simulink model "threeLinks_opt_joint_limit"  (R2016b)
settings: Solver=FixedStepDiscrete  StartTime=0.0  StopTime=inf  FixedStep=Ts  RelTol=1e-3  EnableMultiTasking=on
StartFcn:
  | foundFig=findobj('Tag','trajScope');
  | if ~isempty(foundFig)
  |    close(foundFig);
  | end
undefined symbols (not defined in the file): DiscIntNeverNeededParam, Ts
libraries: simulink x3
settings Model: Creator=pattacini  LastModifiedBy=ben
settings DataIOCC: SaveFormat=Array  SignalLoggingSaveFormat=ModelDataLogs  SaveOutput=off  SignalLogging=off  SaveTime=off
settings OptimizationCC: ExpressionDepthLimit=2147483647  LifeSpan=inf
settings DebuggingCC: UnderspecifiedInitializationDetection=Classic  MergeDetectMultiDrivingBlocksExec=none  SolverPrmCheckMsg=warning  FcnCallInpInsideContextMsg=warning  StateNameClashWarn=warning  SFUnexpectedBacktrackingDiag=warning  SFNoUnconditionalDefaultTransitionDiag=warning  SFExecutionAtInitializationDiag=none
settings HardwareCC: ProdBitPerPointer=32  ProdBitPerSizeT=32  ProdBitPerPtrDiffT=32  ProdLargestAtomicFloat=None  ProdIntDivRoundTo=Undefined  ProdEndianess=Unspecified  ProdWordSize=32  ProdHWDeviceType=32-bit Generic
settings ModelReferenceCC: PropagateSignalLabelsOutOfModel=off
settings SFSimCC: SimParseCustomCode=off
settings GRTTargetCC: TargetLangStandard=C89/C90 (ANSI)  CombineOutputUpdateFcns=off  GRTInterface=on
settings ConfigComp: CovMetricSettings=dw  CovHtmlReporting=on  CovSaveCumulativeToWorkspaceVar=on  CovSaveSingleToWorkspaceVar=on  CovExternalEMLEnable=off

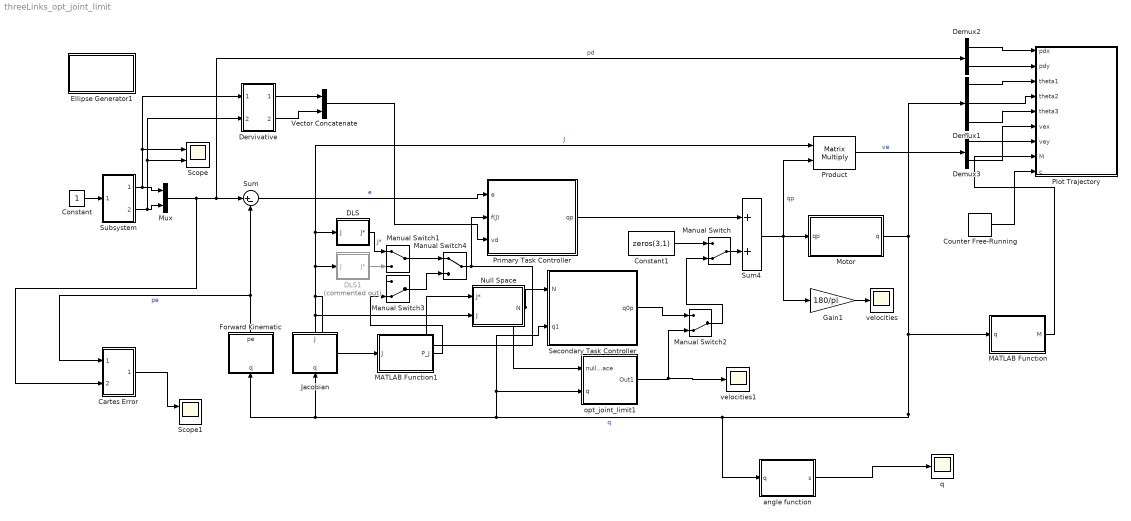
== system threeLinks_opt_joint_limit ==
  Cartes Error : Subsystem
  Constant : Constant
  Constant1 : Constant  Value=zeros(3,1)
  Counter Free-Running : simulink/Sources/Counter Free-Running  NumBits=16  tsamp=-1
  DLS : Subsystem  mask(Motor settings){k=0.01}
      mask Display: port_label('input',1,'DLS');
  DLS1 : Subsystem  Commented=on  mask(Motor settings){W=[4 0 0; 0 1 0; 0 0 1]}
      mask prompts: W "W matrix(3*3)"
      mask Display: port_label('input',1,'W J*');
  Demux1 : Demux  Outputs=3
  Demux2 : Demux  Outputs=2
  Demux3 : Demux  Outputs=2
  Dervivative : Subsystem
  Ellipse Generator1 : Subsystem  mask(Edit sample time){Ts=0.01}
      mask prompts: Ts "Ts [s]:"
      mask init:
      | assignin('base','Ts',Ts);
      mask Display: disp('Edit\nSample Time');
  Forward Kinematic : Subsystem
  Gain1 : Gain  Gain=180/pi
  Jacobian : Subsystem
  MATLAB Function : MATLAB Function  TreatAsAtomicUnit=on
  MATLAB Function1 : MATLAB Function  TreatAsAtomicUnit=on
  Manual Switch : ManualSwitch  CurrentSetting=0
  Manual Switch1 : ManualSwitch
  Manual Switch2 : ManualSwitch  CurrentSetting=0
  Manual Switch3 : ManualSwitch  CurrentSetting=0
  Manual Switch4 : ManualSwitch
  Motor : Subsystem  mask(Motor settings){q0=[pi/4;  pi/4 ;  -pi/4]}
      mask prompts: q0 "Initial position [2x1]:"
      mask Display:
      | disp('Motor');
      | port_label('input',1,'qp');
      | port_label('output',1,'q');
  Mux : Mux  Inputs=2
      settings: DisplayOption=signals
  Null Space : Subsystem
  Plot Trajectory : MATLAB Function  TreatAsAtomicUnit=on
  Primary Task Controller : Subsystem  mask(Controller settings){K=[50 0; 0 50]}
      mask prompts: K "Gain matrix [2x2]:"
      mask Display: disp('qp=J**K*e');
  Product : Product  Multiplication=Matrix(*)  RndMeth=Zero
  Scope : Scope  NumInputPorts=2
  Scope1 : Scope  NumInputPorts=2
  Secondary Task Controller : Subsystem  mask(Controller settings){k=[0 0 1]', q0=[0 0 0]'}
  Subsystem : Subsystem
      mask Display: disp('Input Signal')
  Sum : Sum  Inputs=|+-
  Sum4 : Sum  Inputs=2
  Vector Concatenate : Concatenate
  "angle function " : MATLAB Function  TreatAsAtomicUnit=on
  opt_joint_limit1 : Subsystem  mask{q_min=[-pi;-pi;-pi], q_max=[pi;pi;pi]}
      mask Display: disp('Secondary Task')
  "q " : Scope
  velocities : Scope
  velocities1 : Scope
  wires:
  Jacobian/1(J) -> MATLAB Function1/1(J), DLS1/1(J), Product/1, DLS/1(J), Null Space/2(J)  "J"
  Sum/1 -> Primary Task Controller/1(e)  "e"
  Forward Kinematic/1(pe) -> Cartes Error/1(In1), Sum/2  "pe"
  Mux/1 -> Cartes Error/2(In2), Sum/1, Demux2/1  "pd"
  Sum4/1 -> Product/2, Gain1/1, Motor/1(qp)  "qp"
  Motor/1(q) -> Demux1/1, "angle function "/1(q), opt_joint_limit1/2(q), Secondary Task Controller/2(q1), Forward Kinematic/1(q), Jacobian/1(q), MATLAB Function/1(q)  "q"
  Demux2/1 -> Plot Trajectory/1(pdx)
  Demux2/2 -> Plot Trajectory/2(pdy)
  Demux1/1 -> Plot Trajectory/3(theta1)
  Demux1/2 -> Plot Trajectory/4(theta2)
  Demux3/1 -> Plot Trajectory/6(vex)
  Demux3/2 -> Plot Trajectory/7(vey)
  Product/1 -> Demux3/1  "ve"
  Gain1/1 -> velocities/1
  Demux1/3 -> Plot Trajectory/5(theta3)
  Primary Task Controller/1(qp) -> Sum4/1
  Manual Switch/1 -> Sum4/2
  Constant1/1 -> Manual Switch/1
  Constant/1 -> Subsystem/1(In1)
  Subsystem/1(Out1) -> Dervivative/1(In1), Scope/1, Mux/1
  Subsystem/2(Out2) -> Dervivative/2(In2), Scope/2, Mux/2
  Dervivative/1(Out1) -> Vector Concatenate/1
  Dervivative/2(Out2) -> Vector Concatenate/2
  Vector Concatenate/1 -> Primary Task Controller/3(vd)
  DLS1/1(J*) -> Manual Switch1/2
  DLS/1(J*) -> Manual Switch1/1  "J*"
  Cartes Error/1(Out2) -> Scope1/1
  Null Space/1(N) -> opt_joint_limit1/1(nullspace), Secondary Task Controller/1(N)
  Secondary Task Controller/1(q0p) -> Manual Switch2/1
  Manual Switch2/1 -> Manual Switch/2
  MATLAB Function/1(M) -> Plot Trajectory/8(M)
  Counter Free-Running/1 -> Plot Trajectory/9(c)
  opt_joint_limit1/1(Out1) -> velocities1/1, Manual Switch2/2
  "angle function "/1(s) -> "q "/1
  MATLAB Function1/1(P_J) -> Manual Switch3/2
  Manual Switch3/1 -> Manual Switch4/2
  Manual Switch1/1 -> Manual Switch4/1
  Manual Switch4/1 -> Primary Task Controller/2(f(J)), Null Space/1(J*)

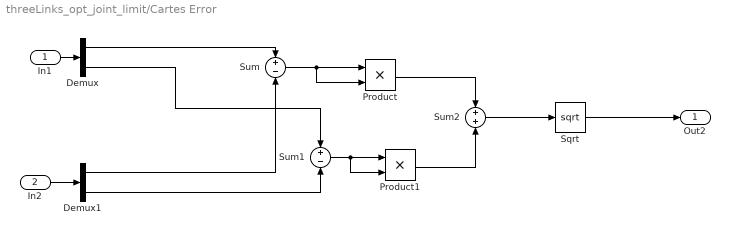
== system threeLinks_opt_joint_limit/Cartes Error ==
  In1 : Inport
  In2 : Inport  Port=2
  Demux : Demux  Outputs=2
  Demux1 : Demux  Outputs=2
  Product : Product
  Product1 : Product
  Sqrt : Sqrt  SaturateOnIntegerOverflow=on
  Sum : Sum  Inputs=+-
  Sum1 : Sum  Inputs=+-
  Sum2 : Sum
  Out2 : Outport
  wires:
  In1/1 -> Demux/1
  In2/1 -> Demux1/1
  Demux/1 -> Sum/1
  Demux1/1 -> Sum/2
  Demux/2 -> Sum1/1
  Demux1/2 -> Sum1/2
  Sum/1 -> Product/2, Product/1
  Sum1/1 -> Product1/2, Product1/1
  Product/1 -> Sum2/1
  Product1/1 -> Sum2/2
  Sum2/1 -> Sqrt/1
  Sqrt/1 -> Out2/1

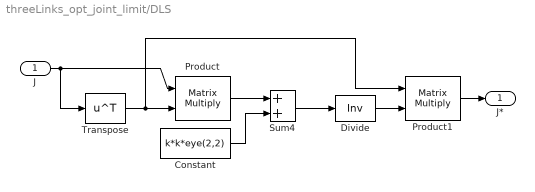
== system threeLinks_opt_joint_limit/DLS ==
  J : Inport
  Constant : Constant  Value=k*k*eye(2,2)
  Divide : Product  Inputs=/  Multiplication=Matrix(*)
  Product : Product  Multiplication=Matrix(*)  RndMeth=Zero
  Product1 : Product  Multiplication=Matrix(*)  RndMeth=Zero
  Sum4 : Sum
  Transpose : Math  Operator=transpose  SaturateOnIntegerOverflow=on
  J* : Outport
  wires:
  J/1 -> Transpose/1, Product/1
  Transpose/1 -> Product/2, Product1/1
  Product/1 -> Sum4/1
  Sum4/1 -> Divide/1
  Divide/1 -> Product1/2
  Product1/1 -> J*/1
  Constant/1 -> Sum4/2

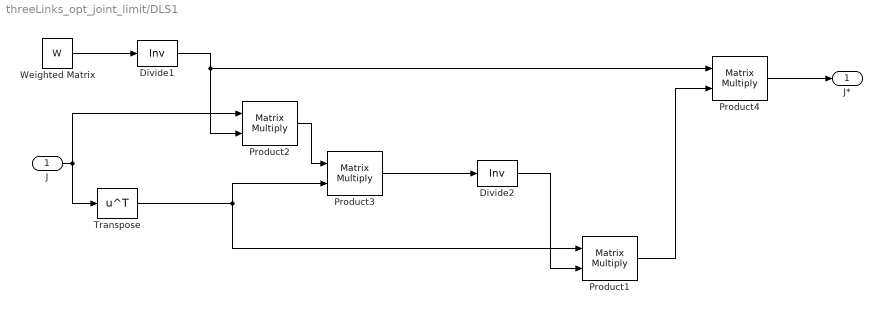
== system threeLinks_opt_joint_limit/DLS1 ==
  J : Inport
  Divide1 : Product  Inputs=/  Multiplication=Matrix(*)
  Divide2 : Product  Inputs=/  Multiplication=Matrix(*)
  Product{1..4} (4 alike) : Product  Multiplication=Matrix(*)  RndMeth=Zero
  Transpose : Math  Operator=transpose  SaturateOnIntegerOverflow=on
  Weighted Matrix : Constant  Value=W
  J* : Outport
  wires:
  J/1 -> Transpose/1, Product2/1
  Weighted Matrix/1 -> Divide1/1
  Divide1/1 -> Product2/2, Product4/1
  Transpose/1 -> Product1/1, Product3/2
  Product2/1 -> Product3/1
  Product3/1 -> Divide2/1
  Product4/1 -> J*/1
  Divide2/1 -> Product1/2
  Product1/1 -> Product4/2

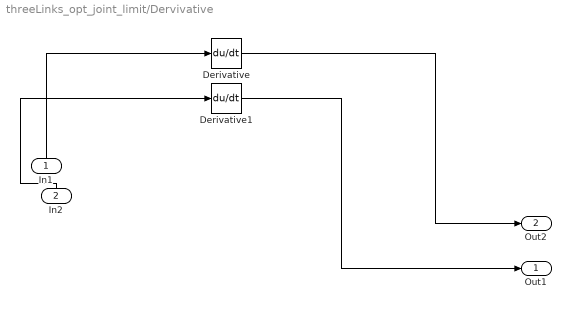
== system threeLinks_opt_joint_limit/Dervivative ==
  In1 : Inport
  In2 : Inport  Port=2
  Derivative : Derivative
  Derivative1 : Derivative
  Out1 : Outport
  Out2 : Outport  Port=2
  wires:
  Derivative/1 -> Out2/1
  In1/1 -> Derivative/1
  Derivative1/1 -> Out1/1
  In2/1 -> Derivative1/1

== system threeLinks_opt_joint_limit/Ellipse Generator1 ==

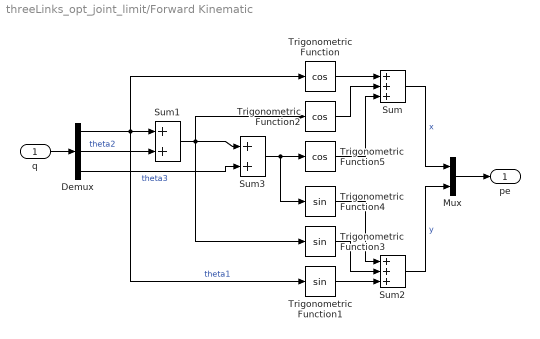
== system threeLinks_opt_joint_limit/Forward Kinematic ==
  q : Inport
  Demux : Demux  Outputs=3
  Mux : Mux  Inputs=2
  Sum : Sum  Inputs=3
  Sum1 : Sum
  Sum2 : Sum  Inputs=3
  Sum3 : Sum
  Trigonometric Function : Trigonometry  Operator=cos
  Trigonometric Function1 : Trigonometry
  Trigonometric Function2 : Trigonometry  Operator=cos
  Trigonometric Function3 : Trigonometry
  Trigonometric Function4 : Trigonometry
  Trigonometric Function5 : Trigonometry  Operator=cos
  pe : Outport
  wires:
  q/1 -> Demux/1
  Demux/1 -> Trigonometric Function1/1, Trigonometric Function/1, Sum1/1  "theta1"
  Mux/1 -> pe/1
  Sum1/1 -> Trigonometric Function2/1, Trigonometric Function3/1, Sum3/1
  Demux/2 -> Sum1/2  "theta2"
  Trigonometric Function1/1 -> Sum2/3
  Trigonometric Function3/1 -> Sum2/2
  Trigonometric Function/1 -> Sum/1
  Trigonometric Function2/1 -> Sum/2
  Demux/3 -> Sum3/2  "theta3"
  Sum3/1 -> Trigonometric Function5/1, Trigonometric Function4/1
  Trigonometric Function5/1 -> Sum/3
  Trigonometric Function4/1 -> Sum2/1
  Sum/1 -> Mux/1  "x"
  Sum2/1 -> Mux/2  "y"

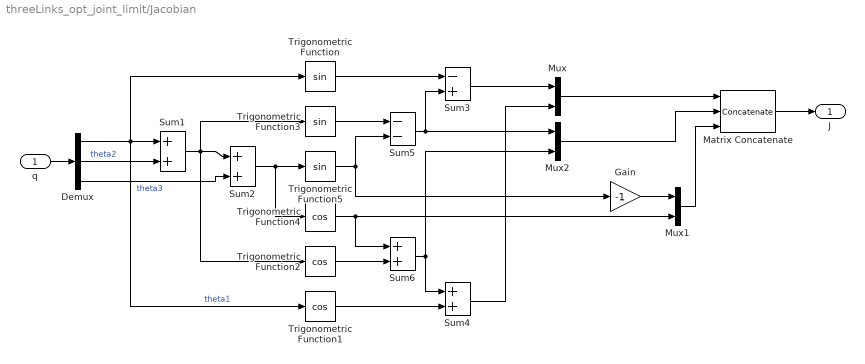
== system threeLinks_opt_joint_limit/Jacobian ==
  q : Inport
  Demux : Demux  Outputs=3
  Gain : Gain  Gain=-1
  Matrix Concatenate : Concatenate  NumInputs=3  Mode=Multidimensional array  ConcatenateDimension=2
  Mux : Mux  Inputs=2
  Mux1 : Mux  Inputs=2
  Mux2 : Mux  Inputs=2
  Sum1 : Sum
  Sum2 : Sum
  Sum3 : Sum  Inputs=-+
  Sum4 : Sum  Inputs=2
  Sum5 : Sum  Inputs=--
  Sum6 : Sum  Inputs=2
  Trigonometric Function : Trigonometry
  Trigonometric Function1 : Trigonometry  Operator=cos
  Trigonometric Function2 : Trigonometry  Operator=cos
  Trigonometric Function3 : Trigonometry
  Trigonometric Function4 : Trigonometry  Operator=cos
  Trigonometric Function5 : Trigonometry
  J : Outport
  wires:
  Demux/1 -> Trigonometric Function/1, Trigonometric Function1/1, Sum1/1  "theta1"
  q/1 -> Demux/1
  Matrix Concatenate/1 -> J/1
  Demux/2 -> Sum1/2  "theta2"
  Sum1/1 -> Trigonometric Function2/1, Trigonometric Function3/1, Sum2/1
  Gain/1 -> Mux1/1
  Demux/3 -> Sum2/2  "theta3"
  Sum2/1 -> Trigonometric Function5/1, Trigonometric Function4/1
  Sum3/1 -> Mux/1
  Sum4/1 -> Mux/2
  Trigonometric Function3/1 -> Sum5/1
  Trigonometric Function5/1 -> Gain/1, Sum5/2
  Sum5/1 -> Sum3/2, Mux2/1
  Trigonometric Function/1 -> Sum3/1
  Trigonometric Function2/1 -> Sum6/2
  Trigonometric Function4/1 -> Mux1/2, Sum6/1
  Trigonometric Function1/1 -> Sum4/2
  Sum6/1 -> Sum4/1, Mux2/2
  Mux/1 -> Matrix Concatenate/1
  Mux2/1 -> Matrix Concatenate/2
  Mux1/1 -> Matrix Concatenate/3

== system threeLinks_opt_joint_limit/Motor ==
  qp : Inport
  Discrete-Time Integrator : DiscreteIntegrator  IntegratorMethod=Integration: Trapezoidal  InitialCondition=q0  SampleTime=Ts  ICPrevOutput=DiscIntNeverNeededParam  ICPrevScaledInput=DiscIntNeverNeededParam
  Unit Delay : UnitDelay  InitialCondition=q0  SampleTime=-1
  q : Outport
  wires:
  qp/1 -> Discrete-Time Integrator/1
  Discrete-Time Integrator/1 -> Unit Delay/1
  Unit Delay/1 -> q/1

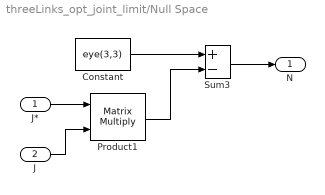
== system threeLinks_opt_joint_limit/Null Space ==
  J* : Inport
  J : Inport  Port=2
  Constant : Constant  Value=eye(3,3)
  Product1 : Product  Multiplication=Matrix(*)  RndMeth=Zero
  Sum3 : Sum  Inputs=+-
  N : Outport
  wires:
  J*/1 -> Product1/1
  J/1 -> Product1/2
  Constant/1 -> Sum3/1
  Product1/1 -> Sum3/2
  Sum3/1 -> N/1

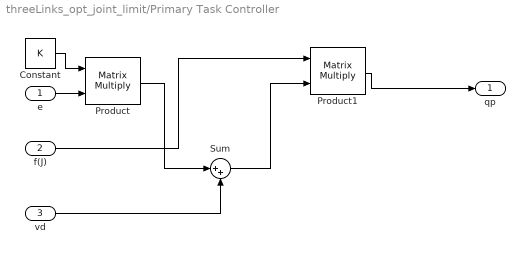
== system threeLinks_opt_joint_limit/Primary Task Controller ==
  e : Inport
  f(J) : Inport  Port=2
  vd : Inport  Port=3
  Constant : Constant  Value=K
  Product : Product  Multiplication=Matrix(*)  RndMeth=Zero
  Product1 : Product  Multiplication=Matrix(*)  RndMeth=Zero
  Sum : Sum  Inputs=|++
  qp : Outport
  wires:
  f(J)/1 -> Product1/1
  e/1 -> Product/2
  Constant/1 -> Product/1
  Product/1 -> Sum/1
  Product1/1 -> qp/1
  vd/1 -> Sum/2
  Sum/1 -> Product1/2

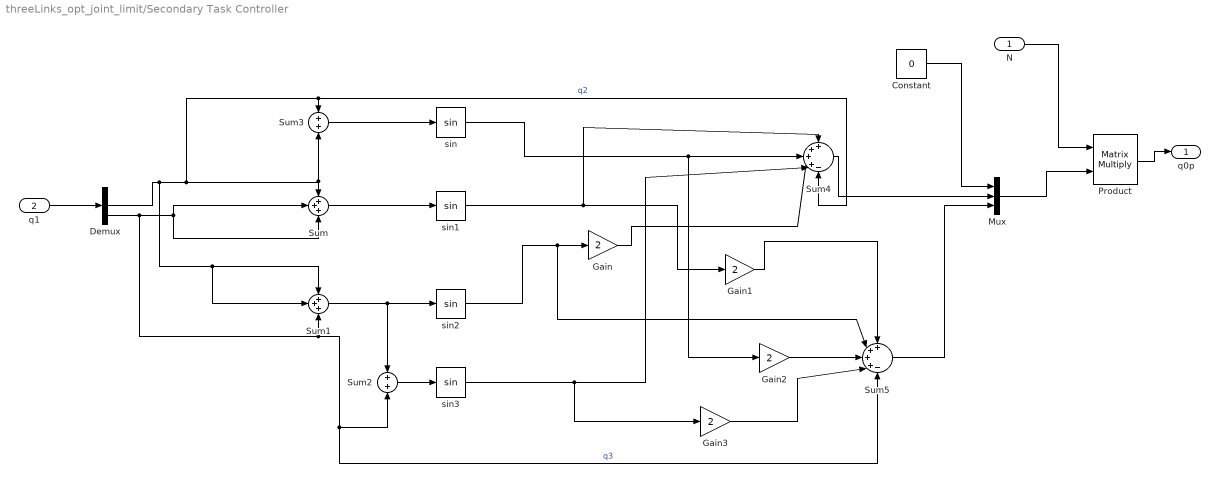
== system threeLinks_opt_joint_limit/Secondary Task Controller ==
  N : Inport
  q1 : Inport  Port=2
  Constant : Constant  Value=0
  Demux : Demux  Outputs=3
  Gain{,1..3} (4 alike) : Gain  Gain=2
  Mux : Mux  Inputs=3
  Product : Product  Multiplication=Matrix(*)
  Sum : Sum  Inputs=+++
  Sum1 : Sum  Inputs=+++
  Sum2 : Sum
  Sum3 : Sum
  Sum4 : Sum  Inputs=++++-
  Sum5 : Sum  Inputs=++++-
  sin{,1..3} (4 alike) : Trigonometry
  q0p : Outport
  wires:
  Demux/2 -> Sum1/2, Sum1/1, Sum4/5, Sum3/1, Sum3/2, Sum/1  "q2"
  Demux/3 -> Sum/3, Sum/2, Sum5/5, Sum2/2, Sum1/3  "q3"
  Sum1/1 -> Sum2/1, sin2/1
  Sum2/1 -> sin3/1
  Sum/1 -> sin1/1
  Sum3/1 -> sin/1
  sin1/1 -> Gain1/1, Sum4/1
  sin2/1 -> Gain/1, Sum5/2
  Gain/1 -> Sum4/2
  sin/1 -> Gain2/1, Sum4/3
  sin3/1 -> Gain3/1, Sum4/4
  Gain1/1 -> Sum5/1
  Gain2/1 -> Sum5/3
  Gain3/1 -> Sum5/4
  Sum4/1 -> Mux/2
  Sum5/1 -> Mux/3
  Constant/1 -> Mux/1
  q1/1 -> Demux/1
  N/1 -> Product/1
  Mux/1 -> Product/2
  Product/1 -> q0p/1

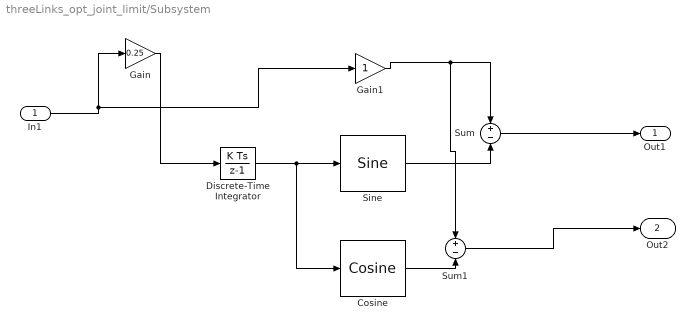
== system threeLinks_opt_joint_limit/Subsystem ==
  In1 : Inport
  Cosine : simulink/Lookup Tables/Cosine  Formula=cos(2*pi*u)  NumDataPoints=(2^5)+1  OutputWordLength=16  InternalRulePriority=Speed
  Discrete-Time Integrator : DiscreteIntegrator  gainval=0.5  InitialConditionSetting=State (most efficient)  SampleTime=Ts  ICPrevOutput=DiscIntNeverNeededParam  ICPrevScaledInput=DiscIntNeverNeededParam
  Gain : Gain  Gain=0.25
  Gain1 : Gain
  Sine : simulink/Lookup Tables/Sine  Formula=sin(2*pi*u)  NumDataPoints=(2^5)+1  OutputWordLength=16  InternalRulePriority=Speed
  Sum : Sum  Inputs=+-
  Sum1 : Sum  Inputs=+-
  Out1 : Outport
  Out2 : Outport  Port=2
  wires:
  In1/1 -> Gain1/1, Gain/1
  Sum1/1 -> Out2/1
  Discrete-Time Integrator/1 -> Cosine/1, Sine/1
  Gain/1 -> Discrete-Time Integrator/1
  Sine/1 -> Sum/2
  Sum/1 -> Out1/1
  Cosine/1 -> Sum1/2
  Gain1/1 -> Sum1/1, Sum/1

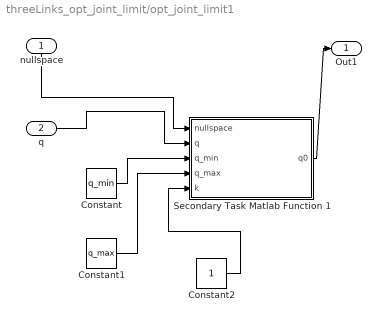
== system threeLinks_opt_joint_limit/opt_joint_limit1 ==
  nullspace : Inport
  q : Inport  Port=2
  Constant : Constant  Value=q_min
  Constant1 : Constant  Value=q_max
  Constant2 : Constant
  Secondary Task Matlab Function 1 : MATLAB Function  TreatAsAtomicUnit=on
  Out1 : Outport
  wires:
  nullspace/1 -> Secondary Task Matlab Function 1/1(nullspace)
  q/1 -> Secondary Task Matlab Function 1/2(q)
  Secondary Task Matlab Function 1/1(q0) -> Out1/1
  Constant1/1 -> Secondary Task Matlab Function 1/4(q_max)
  Constant/1 -> Secondary Task Matlab Function 1/3(q_min)
  Constant2/1 -> Secondary Task Matlab Function 1/5(k)

== matlab function threeLinks_opt_joint_limit/MATLAB Function ==
  data: q input; M output
function M = v_ellipse(q)
%#codegen
 M = [                       sin(q(1) + q(2) + q(3))^2 + (sin(q(1) + q(2) + q(3)) + sin(q(1) + q(2)) + sin(q(1)))^2 + (sin(q(1) + q(2) + q(3)) + sin(q(1) + q(2)))^2, - sin(2*q(1) + q(2)) - sin(2*q(1))/2 - (3*sin(2*q(1) + 2*q(2) + 2*q(3)))/2 - sin(2*q(1) + 2*q(2)) - sin(2*q(1) + q(2) + q(3)) - 2*sin(2*q(1) + 2*q(2) + q(3));...
     - sin(2*q(1) + q(2)) - sin(2*q(1))/2 - (3*sin(2*q(1) + 2*q(2) + 2*q(3)))/2 - sin(2*q(1) + 2*q(2)) - sin(2*q(1) + q(2) + q(3)) - 2*sin(2*q(1) + 2*q(2) + q(3)),                       (cos(q(1) + q(2) + q(3)) + cos(q(1) + q(2)) + cos(q(1)))^2 + cos(q(1) + q(2) + q(3))^2 + (cos(q(1) + q(2) + q(3)) + cos(q(1) + q(2)))^2]

== matlab function threeLinks_opt_joint_limit/angle function  ==
  data: q input; s output
function s = angle(q)
    q_o = zeros(3,1)
    q_o(1,:) = mod((q(1)*180/pi+180),360)- 180;
    q_o(2,:) = mod((q(2)*180/pi+180),360)- 180;
    q_o(3,:) = mod((q(3)*180/pi+180),360)- 180;
    s = norm(q_o)

== matlab function threeLinks_opt_joint_limit/Plot Trajectory ==
  data: pdx input; pdy input; theta1 input; theta2 input; theta3 input; vex input; vey input; M input; c input
function PlotTraj(pdx,pdy,theta1,theta2,theta3,vex,vey,M,c)
% Author: Ugo Pattacini

coder.extrinsic('findobj','get','set','figure','clf',...
              'hold','delete','plot','axis','grid',...
              'hggroup','quiver','drawnow');
          
persistent target;
persistent chain;
  
pex=[0;...
    cos(theta1);...
    cos(theta1)+cos(theta1+theta2);...
    cos(theta1)+cos(theta1+theta2)+cos(theta1+theta2+theta3)];

pey=[0;...
    sin(theta1);...
    sin(theta1)+sin(theta1+theta2);...
    sin(theta1)+sin(theta1+theta2)+sin(theta1+theta2+theta3)];
          
foundFig=findobj('Tag','trajScope');

if isempty(foundFig)
    fig=figure('Color','white');
    clf(fig);
    set(fig,'Name','Trajectory');
    set(fig,'DoubleBuffer','on','Tag','trajScope');
    set(fig,'Renderer','painters');
    hold('on');
    hax=get(fig,'CurrentAxes');
    set(hax,'DrawMode','fast','Box','off');    
    
    target=plot(hax,pdx,pdy,'bo','MarkerFaceColor','b');

    chain=hggroup;
    h1=plot(hax,pex,pey,'r','LineWidth',3);
    h2=plot(hax,pex(1),pey(1),'ro','MarkerFaceColor','r');
    h3=plot(hax,pex(2),pey(2),'ro','MarkerFaceColor','r');
    h4=plot(hax,pex(3),pey(3),'ro','MarkerFaceColor','r');
    h5=plot(hax,pex(4),pey(4),'ro','MarkerFaceColor','r');
    set(h1,'Parent',chain);
    set(h2,'Parent',chain);
    set(h3,'Parent',chain);
    set(h4,'Parent',chain);
    set(h5,'Parent',chain);
    
    


    axis([-3.3 3.3 -3.3 3.3]);
    axis('equal');
    grid('on');
else    
    hax=get(foundFig,'CurrentAxes');
end

if ~isempty(chain)
    delete(target);
    delete(chain);
end


% draw the desired point
target=plot(hax,pdx,pdy,'bo','MarkerFaceColor','b');

% draw the link
chain=hggroup;
h1=plot(hax,pex,pey,'r','LineWidth',3);
h2=plot(hax,pex(1),pey(1),'ro','MarkerFaceColor','r');
h3=plot(hax,pex(2),pey(2),'ro','MarkerFaceColor','r');
h4=plot(hax,pex(3),pey(3),'ro','MarkerFaceColor','r');
h5=plot(hax,pex(4),pey(4),'ro','MarkerFaceColor','r');
set(h1,'Parent',chain);
set(h2,'Parent',chain);
set(h3,'Parent',chain);
set(h4,'Parent',chain);
set(h5,'Parent',chain);

% draw the end-effector velocity in the cartesian space
%velocity=quiver(hax,pex(end),pey(end),vex,vey,'Color','green','LineWidth',2);



if (mod(c,200)==1) & (c/200>0)
    hold on
    plot(hax,pdx,pdy,'-.ko','MarkerFaceColor','k');

    % draw the link
    plot(hax,pex,pey,'k','LineWidth',1);
    plot(hax,pex(1),pey(1),':ko','MarkerFaceColor','k');
    plot(hax,pex(2),pey(2),':ko','MarkerFaceColor','k');
    plot(hax,pex(3),pey(3),':ko','MarkerFaceColor','k');
    plot(hax,pex(4),pey(4),':ko','MarkerFaceColor','k');


    % draw the end-effector velocity in the cartesian space
    %velocity=quiver(hax,pex(end),pey(end),vex,vey,'Color','green','LineWidth',2);

 
end

drawnow;

== matlab function threeLinks_opt_joint_limit/MATLAB Function1 ==
  data: J input; P_J output
function P_J = p_J(J)
    P_J = J.'*inv(J*J.')

== matlab function threeLinks_opt_joint_limit/opt_joint_limit1/Secondary Task Matlab Function 1 ==
  data: nullspace input; q0 output; q input; q_min input; q_max input; k input
function q0 = f_q0(nullspace,q,q_min,q_max,k)
%#codegen

q_0 =  [-(4*q_min(1) - 8*q(1) + 4*q_max(1))/(24*(q_min(1) - q_max(1))^2);...
        -(4*q_min(2) - 8*q(2) + 4*q_max(2))/(24*(q_min(2) - q_max(2))^2);...
        -(4*q_min(3) - 8*q(3) + 4*q_max(3))/(24*(q_min(3) - q_max(3))^2)]
q_0 = [-q(1);-q(2);-q(3)]
q_0 = q_0/norm(q_0)
q_0 = k*q_0


    
q0 = nullspace*q_0
